simulink model "DSB"  (R2020b)
settings: Solver=VariableStepAuto  StartTime=0.0  StopTime=1  RelTol=1e-3
libraries: dsparch4 x1
settings Model: Creator=LENOVO  LastModifiedBy=LENOVO

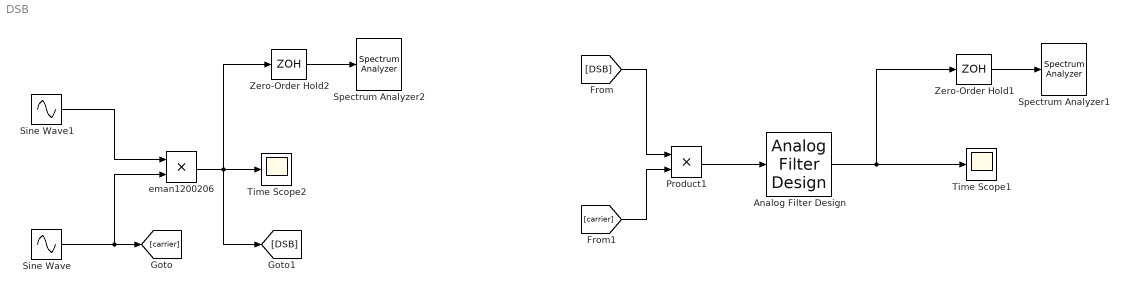
== system DSB ==
  Analog Filter Design : dsparch4/Analog Filter Design  method=Butterworth  filttype=Lowpass  N=2  Wlo=2*pi*1000  Whi=80  Rp=2  Rs=40
  Product1 : Product
  Sine Wave : Sin  Frequency=2*pi*15000  Phase=2*pi*90  SampleTime=0
  Sine Wave1 : Sin  Amplitude=0.85  Frequency=2*pi*1000  Phase=2*pi*90  SampleTime=0
  Spectrum Analyzer1 : SpectrumAnalyzer
  Spectrum Analyzer2 : SpectrumAnalyzer
  Time Scope1 : Scope
  Time Scope2 : Scope
  Zero-Order Hold1 : ZeroOrderHold  SampleTime=-1
  Zero-Order Hold2 : ZeroOrderHold  SampleTime=-1
  eman1200206 : Product
  wires:
  [DSB] -> Product1/1
  [carrier] -> Product1/2
  Product1/1 -> Analog Filter Design/1
  Analog Filter Design/1 -> Zero-Order Hold1/1, Time Scope1/1
  Zero-Order Hold1/1 -> Spectrum Analyzer1/1
  Sine Wave1/1 -> eman1200206/1
  Sine Wave/1 -> [carrier], eman1200206/2
  eman1200206/1 -> Zero-Order Hold2/1, [DSB], Time Scope2/1
  Zero-Order Hold2/1 -> Spectrum Analyzer2/1
